simulink model "Sim01"  (R2019a)
settings: Solver=VariableStepAuto  StartTime=0.0  StopTime=10.0  MaxStep=0.001  RelTol=1e-3
settings Model: Creator=Administrator  LastModifiedBy=Cybaster
settings DataIOCC: ReturnWorkspaceOutputs=off
settings DebuggingCC: ArithmeticOperatorsInVariantConditions=warning

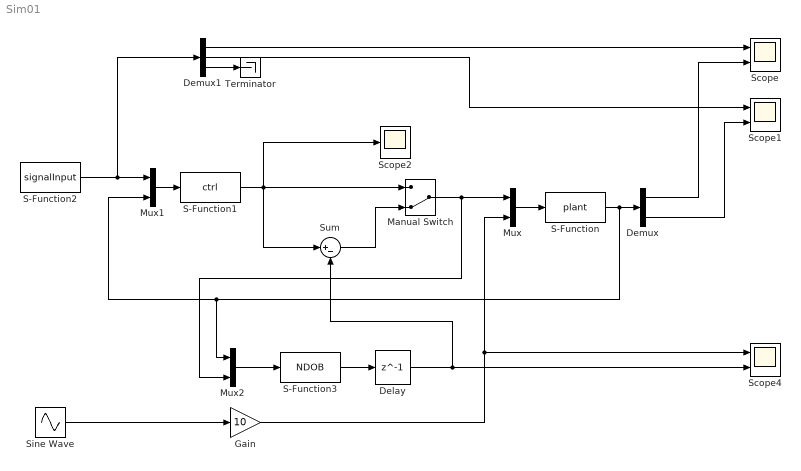
== system Sim01 ==
  Delay : Delay  DelayLength=1  InitialCondition=0
  Demux : Demux  Outputs=2
  Demux1 : Demux  Outputs=3
  Gain : Gain  Gain=10
  Manual Switch : ManualSwitch  CurrentSetting=0
  Mux : Mux  Inputs=2
  Mux1 : Mux  Inputs=2
  Mux2 : Mux  Inputs=2
  S-Function : S-Function  FunctionName=plant  SFunctionDeploymentMode=off  EnableBusSupport=off
  S-Function1 : S-Function  FunctionName=ctrl  SFunctionDeploymentMode=off  EnableBusSupport=off
  S-Function2 : S-Function  FunctionName=signalInput  SFunctionDeploymentMode=off  EnableBusSupport=off
  S-Function3 : S-Function  FunctionName=NDOB  SFunctionDeploymentMode=off  EnableBusSupport=off
  Scope : Scope  NumInputPorts=2
  Scope1 : Scope  NumInputPorts=2
  Scope2 : Scope
  Scope4 : Scope  NumInputPorts=2
  Sine Wave : Sin  SampleTime=0
  Sum : Sum  Inputs=|+-
  Terminator : Terminator
  wires:
  Mux/1 -> S-Function/1
  Sine Wave/1 -> Gain/1
  S-Function1/1 -> Sum/1, Manual Switch/1, Scope2/1
  Mux1/1 -> S-Function1/1
  S-Function2/1 -> Demux1/1, Mux1/1
  S-Function/1 -> Demux/1, Mux2/1, Mux1/2
  Demux/1 -> Scope/2
  Demux1/1 -> Scope/1
  Demux1/2 -> Scope1/1
  Demux/2 -> Scope1/2
  Mux2/1 -> S-Function3/1
  S-Function3/1 -> Delay/1
  Manual Switch/1 -> Mux/1, Mux2/2
  Sum/1 -> Manual Switch/2
  Demux1/3 -> Terminator/1
  Gain/1 -> Mux/2, Scope4/1
  Delay/1 -> Sum/2, Scope4/2
